simulink model "Control_IBA_ACT"  (R2023b)
settings: Solver=VariableStepAuto  StartTime=0.0  StopTime=inf  RelTol=1e-3
settings Model: Creator=Alberto  LastModifiedBy=Alberto

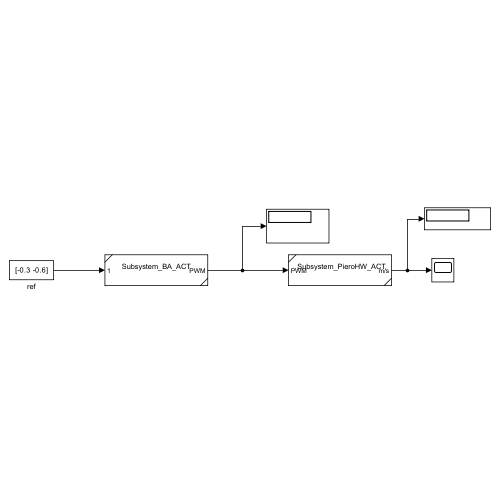
[thumbnail: Simulink's stored preview of the top-level diagram]
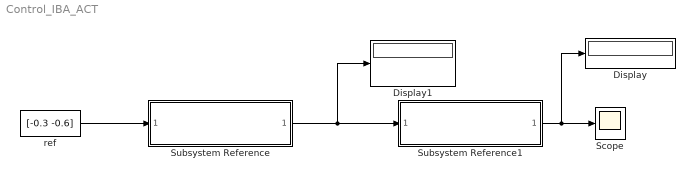
== system Control_IBA_ACT ==
  Display : Display
  Display1 : Display
  Scope : Scope
  Subsystem Reference : Subsystem  ReferencedSubsystem=Subsystem_BA_ACT
  Subsystem Reference1 : Subsystem  ReferencedSubsystem=Subsystem_PieroHW_ACT
  ref : Constant  Value=[-0.3 -0.6]
  wires:
  ref/1 -> Subsystem Reference/1
  Subsystem Reference/1 -> Display1/1, Subsystem Reference1/1
  Subsystem Reference1/1 -> Display/1, Scope/1
